simulink model "A"  (R2021a)
settings: Solver=VariableStepAuto  StartTime=0.0  StopTime=10.0  RelTol=1e-3
libraries: simulink_extras x5, spsSeriesRLCBranchLib x4, spsDCVoltageSourceLib x1, spsVoltageMeasurementLib x1, spspowerguiLib x1
settings Model: Creator=solo  LastModifiedBy=solo

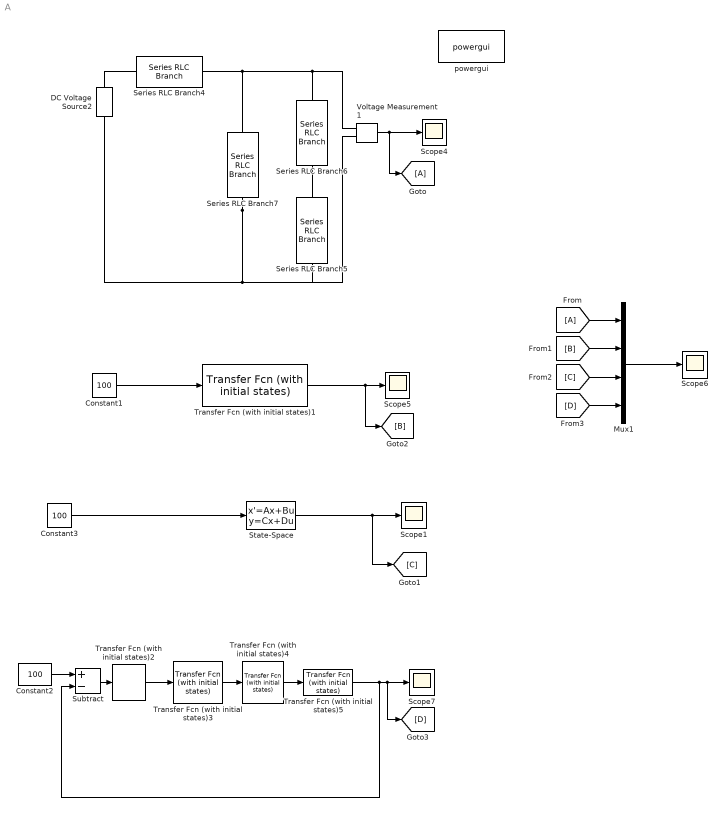
== system A ==
  Constant1 : Constant  Value=100
  Constant2 : Constant  Value=100
  Constant3 : Constant  Value=100
  DC Voltage Source2 : spsDCVoltageSourceLib/DC Voltage Source  Amplitude=100  Measurements=None
  Mux1 : Mux
  Scope{1,4..7} (5 alike) : Scope
  Series RLC Branch4 : spsSeriesRLCBranchLib/Series RLC Branch  LConnTagsString=__new0  RConnTagsString=__new0  BranchType=R  Resistance=1  Inductance=1e-3  SetiL0=off  InitialCurrent=0  Capacitance=1e-6  Setx0=off  InitialVoltage=0  Measurements=None
  Series RLC Branch5 : spsSeriesRLCBranchLib/Series RLC Branch  LConnTagsString=__new0  RConnTagsString=__new0  BranchType=C  Resistance=4  Inductance=1e-3  SetiL0=off  InitialCurrent=0  Capacitance=6  Setx0=on  InitialVoltage=0  Measurements=None
  Series RLC Branch6 : spsSeriesRLCBranchLib/Series RLC Branch  LConnTagsString=__new0  RConnTagsString=__new0  BranchType=R  Resistance=3  Inductance=1e-3  SetiL0=off  InitialCurrent=0  Capacitance=1e-6  Setx0=off  InitialVoltage=0  Measurements=None
  Series RLC Branch7 : spsSeriesRLCBranchLib/Series RLC Branch  LConnTagsString=__new0  RConnTagsString=__new0  BranchType=C  Resistance=4  Inductance=1e-3  SetiL0=off  InitialCurrent=0  Capacitance=5  Setx0=on  InitialVoltage=0  Measurements=None
  State-Space : StateSpace  A="[0  1 ;-1/90  -29/90]"  B="[0  ; 1/90]"  C="[1  18]"  D=0  InitialCondition=0
  Subtract : Sum  Inputs=+-
  Transfer Fcn (with initial states)1 : simulink_extras/Additional Linear/Transfer Fcn (with initial states)  N=[18 1]  D=[90 29 1]  X0=0
  Transfer Fcn (with initial states)2 : simulink_extras/Additional Linear/Transfer Fcn (with initial states)  N=[1]  D=[ 1]  X0=0
  Transfer Fcn (with initial states)3 : simulink_extras/Additional Linear/Transfer Fcn (with initial states)  N=[1]  D=[ 5 0]  X0=0
  Transfer Fcn (with initial states)4 : simulink_extras/Additional Linear/Transfer Fcn (with initial states)  N=[18 1]  D=[6 0]  X0=0
  Transfer Fcn (with initial states)5 : simulink_extras/Additional Linear/Transfer Fcn (with initial states)  N=[30 0 0]  D=[90 11 0]  X0=0
  Voltage Measurement1 : spsVoltageMeasurementLib/Voltage Measurement  PhasorSimulation=off  OutputType=Complex  PSBequivalent=0
  powergui : spspowerguiLib/powergui  Priority=1  SimulationMode=Continuous  SampleTime=50e-6  frequency=60  Iterations=50  frequencyindice=0  Pbase=100e6  ErrMax=1e-4  UnitsV=kV  UnitsW=MW  buscounter=0  FunctionMessages=off  echomessages=off  EnableUseOfTLC=off  CurrentSourceSwitches=off  DisableSnubberDevices=off  DisableRonSwitches=off  DisableVfSwitches=off  DisplayEquations=off  AutomaticDiscreteSolvers=off  SolverType=Tustin/Backward Euler (TBE)  Interpol=off  ExternalGateDelay=off  methode=off  Ts=100  x0status=blocks  SPID=on  SwTol=0  HookPort=off  NonlinearTolerance=1e-4  nMaxIteration=100  ContinueOnMaxIteration=off  RestoreLinks=warning  ResistiveCurrentMeasurement=off  Frange=[0:2:500]  Ylog=off  Xlog=on  ShowGrid=off  save=off  variable=ZData  structure=0  ZoomFFT=off  StartTime=0.0  cycles=1  DisplayStyle=1  fundamental=60  FreqAxis=off  MaxFrequency=1000  frequencyindicesteady=1  RmsSteady=1  display=off
  wires:
  Transfer Fcn (with initial states)2/1 -> Transfer Fcn (with initial states)3/1
  [A] -> Mux1/1
  [C] -> Mux1/3
  [D] -> Mux1/4
  Transfer Fcn (with initial states)1/1 -> [B], Scope5/1
  Constant2/1 -> Subtract/1
  Transfer Fcn (with initial states)5/1 -> Subtract/2, [D], Scope7/1
  Constant3/1 -> State-Space/1
  Subtract/1 -> Transfer Fcn (with initial states)2/1
  Transfer Fcn (with initial states)3/1 -> Transfer Fcn (with initial states)4/1
  State-Space/1 -> [C], Scope1/1
  Constant1/1 -> Transfer Fcn (with initial states)1/1
  Transfer Fcn (with initial states)4/1 -> Transfer Fcn (with initial states)5/1
  Voltage Measurement1/1 -> [A], Scope4/1
  [B] -> Mux1/2
  Mux1/1 -> Scope6/1
  connections:
  Series RLC Branch7/LConn1 -- Series RLC Branch6/LConn1 -- Voltage Measurement1/LConn1 -- Series RLC Branch4/RConn1
  Series RLC Branch7/RConn1 -- Series RLC Branch5/RConn1 -- Voltage Measurement1/LConn2 -- DC Voltage Source2/LConn1
  DC Voltage Source2/RConn1 -- Series RLC Branch4/LConn1
  Series RLC Branch5/LConn1 -- Series RLC Branch6/RConn1
